simulink model "model_tlc"  (Simulink 7.5)
settings: Solver=ode45  StartTime=0.0  StopTime=inf  RelTol=1e-3
settings Model: Creator=paris  LastModifiedBy=paris

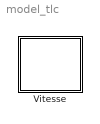
== system model_tlc ==
  Vitesse : Stateflow chart  TreatAsAtomicUnit=on

== stateflow chart Vitesse ==
  state lent
  state rapide
  (default) -> lent
  lent -> rapide : [ml.vitesse>=30]
  rapide -> lent : [ml.vitesse<30]
